simulink library "sensor_library"  (R2018b)
settings: Solver=VariableStepAuto  StartTime=0.0  StopTime=10.0  RelTol=1e-3
undefined symbols (not defined in the file): DiscIntNeverNeededParam, EOP_IERS, GPS, GPS_sensor_time, GYRO, GYRO_sensor_time, jdate0
libraries: dspsigops x26, simulink x9, simulink_extras x4
(part 2 of 2)

== matlab function sensor_library/GPS Model - [m, m//s]/GPS Clock ==
  data: jdutc input; jdut1 output; dut1 input; dat input; utc output; gps_reference output; time_error input; offset output; utc_offset output
%GPS Clock from time_convert
function [jdut1,utc,gps_reference,offset,utc_offset]= time_convert(jdutc, dut1, dat, time_error)

% ---- convert time
% Input Julian is in UTC
% UTC = UT1 - dUT1
% UT1 = UTC + dUT1
% TAI = UTC + dAT
% GPS = TAI - 19s
% TT  = GPS + 19s + 32.184s

% jdut1: is the real time to perform conversion (No error is applied)
% utc: is the estimated utc time [year,mon,day,hr,min,sec] (including time error)
% gps_reference: is the estimated gps reference time (including time error)
% offset: Receiver clock offset in seconds from GPS system time.
% utc_offset: the offset of GPS system time from UTC time, computed using almanac parameters.


% GPS reference time is the receiver’s estimate of the true GPS system time. 
% GPS reference time can be found in the header of the TIME log. 
% The relationship between GPS reference time and true GPS system time is:
% GPS system time = GPS reference time - offset


% UTC time is GPS reference time plus the current UTC offset minus the receiver clock offset
% UTC time = GPS reference time - offset + UTC offset

% ------------------------  implementation   ------------------
jdutcint=fix(jdutc);
jdutfrac=rem(jdutc,1);


%%%%%%%%%%%%%%%%%%%%%% utc
[year,mon,day,hr,min,sec] = invjday_s (jdutcint, jdutfrac);
utc_hms = hms2sec_s(hr, min, sec );

%%%%%%%%%%%%%%%%%%%%%% ut1
ut1_hms= utc_hms + dut1;
[hrtemp,mintemp,sectemp] = sec2hms_s(ut1_hms);
[jdut1int, jdut1frac] = jday_s(year,mon,day, hrtemp, mintemp, sectemp );
jdut1=jdut1int+jdut1frac;

%%%%%%%%%%%%%%%%%%%%%% output utc
utc=[year,mon,day,hr,min,sec+time_error];

%%%%%%%%%%%%%%%%%%%%%% tai
tai_hms= utc_hms + dat + time_error;

%%%%%%%%%%%%%%%%%%%%%% gps
gps_hms= tai_hms - 19; %sec
[hrtemp,mintemp,sectemp] = sec2hms_s(gps_hms);
[jdgpsint, jdgpsfrac] = jday_s(year,mon,day, hrtemp, mintemp, sectemp );
jdgps=jdgpsint+jdgpsfrac;
jdgps0 = 2.444244500000000e+06; %juliandate(1980,1,6);    % beginning of GPS week numbering
nweek = fix((jdgps-jdgps0)/7);
sow = (jdgps - (jdgps0+nweek*7)) * 3600*24;
% check sow
if sow > 604800
    nweek = nweek + 1;
    sow = sow - 604800;
elseif sow < 0
    nweek = nweek - 1;
    sow = sow + 604800;
end
gps_reference=[nweek,sow];

%%%%%%%%%%%%%%%%%%%%%% offset
offset = time_error; %To be calibrated - Now assumed to be equal to time accuracy, in order to retrieve real time
utc_offset= utc_hms - gps_hms + offset;   %UTC offset = UTC time - GPS reference time + offsert 

end

% -----------------------------------------------------------------------------
%
%                           function jday.m
%

function [jd, jdfrac] = jday_s(yr, mon, day, hr, min, sec)

% ------------------------  implementation   ------------------
jd = 367.0 * yr  ...
    - floor( (7 * (yr + floor( (mon + 9) / 12.0) ) ) * 0.25 )   ...
    + floor( 275 * mon / 9.0 ) ...
    + day + 1721013.5;   % use - 678987.0 to go to mjd directly
jdfrac = (sec + min * 60.0 + hr *3600.0) / 86400.0;

% check jdfrac
if jdfrac > 1.0
    jd = jd + floor(jdfrac);
    jdfrac = jdfrac - floor(jdfrac);
end

%  - 0.5 * sign(100.0 * yr + mon - 190002.5) + 0.5;
end

% -----------------------------------------------------------------------------
%
%                           function invjday.m
%


function [year,mon,day,hr,min,sec] = invjday_s (jd, jdfrac)

% check jdfrac for multiple days
if abs(jdfrac) >= 1.0
    jd = jd + floor(jdfrac);
    jdfrac = jdfrac - floor(jdfrac);
end

% check for fraction of a day included in the jd
dt = jd - floor(jd) - 0.5;
if (abs(dt) > 0.00000001)
    jd = jd - dt;
    jdfrac = jdfrac + dt;
end

% ----------------- find year and days of the year ---------------
temp   = jd - 2415019.5;
tu     = temp / 365.25;
year   = 1900 + floor( tu );
leapyrs= floor( ( year-1901 )*0.25 );
days   = floor(temp - ((year-1900)*365.0 + leapyrs ));

% ------------ check for case of beginning of a year -------------
if days + jdfrac < 1.0
    year   = year - 1;
    leapyrs= floor( ( year-1901 )*0.25 );
    days   = floor(temp - ((year-1900)*365.0 + leapyrs ));
end

% ------------------- find remaining data  -----------------------
% now add the daily time in to preserve accuracy
[mon,day,hr,min,sec] = days2mdh_s(year, days + jdfrac);
end

% -----------------------------------------------------------------------------
%
%                           function sec2hms
%
function [hr,min,sec] = sec2hms_s(utsec)

% ------------------------  implementation   ------------------
temp  = utsec / 3600.0;
hr    = fix( temp );
min   = fix( (temp - hr)* 60.0 );
sec   = (temp - hr - min/60.0 ) * 3600.0;
end

% -----------------------------------------------------------------------------
%
%                           function hms2sec
%
function [utsec] = hms2sec_s(hr,min,sec )

% ------------------------  implementation   ------------------
utsec  = hr * 3600.0 + min * 60.0 + sec;

end



% -----------------------------------------------------------------------------
%
%                           function days2mdh
%
function [mon,day,hr,minute,sec] = days2mdh_s (year,days)

% --------------- set up array of days in month  --------------
lmonth=zeros(12,1);
for i= 1 : 12
    lmonth(i) = 31;
    if i == 2
        lmonth(i)= 28;
    end
    if i == 4 || i == 6 || i == 9 || i == 11
        lmonth(i)= 30;
    end
end

dayofyr= floor(days);

% ----------------- find month and day of month ---------------
if rem(year-1900,4) == 0
    lmonth(2)= 29;
end

i= 1;
inttemp= 0;
while ( dayofyr > inttemp + lmonth(i) ) && ( i < 12 )
    inttemp= inttemp + lmonth(i);
    i= i+1;
end

mon= i;
day= dayofyr - inttemp;

% ----------------- find hours minutes and seconds ------------
temp = (days - dayofyr )*24.0;
hr  = fix( temp );
temp = (temp-hr) * 60.0;
minute = fix( temp );
sec = (temp-minute) * 60.0;
end

== matlab function sensor_library/GPS Model - [m, m//s]/ECI to ECEF [m,m//s] ==
  data: reci input; recef output; veci input; jdut1 input; dutt input; lod input; xp input; yp input; ddpsi input; ddeps input; vecef output
% ECI to ECEF from eci2ecef_s
% I/O - [m, m/s]

function [recef,vecef] = eci2ecef_s(reci,veci,jdut1,dutt,lod,xp,yp,ddpsi,ddeps)

eqeterms=2;
reci=reshape(reci,3,1);
veci=reshape(veci,3,1);

% ---- convert time
% Input Julian is in UT1
% UTC = UT1+dUT1
% TAI = UTC + dAT
% TT  = TAI + 32.184s
jdutt=jdut1+(dutt/24/60/60);

% Julian centuries from J2000.0
ttt=(jdutt-2451545.0)/36525;

% ---- find matrices
[prec] = precess_s(ttt);

[deltapsi,~,meaneps,omega,nut] = nutation_s(ttt,ddpsi,ddeps);

[st] = sidereal_s(jdut1,deltapsi,meaneps,omega,eqeterms );

[pm] = polarm_s(xp,yp);

% ---- perform transformations
thetasa= 7.29211514670698e-05 * (1.0  - lod/86400.0 );
omegaearth = [0; 0; thetasa;];

rpef  = st'*nut'*prec'*reci;
recef = pm'*rpef;

vpef  = st'*nut'*prec'*veci - cross( omegaearth,rpef );
vecef = pm'*vpef;

end

% -----------------------------------------------------------------------------
%
%                           function precess

function prec = precess_s (ttt)

prec=zeros(3,3);

% " to rad
convrt = pi / (180.0*3600.0);
ttt2= ttt * ttt;
ttt3= ttt2 * ttt;

% ------------------- fk4 b1980 precession angles --------------------
zeta =             2306.2181*ttt + 0.30188*ttt2 + 0.017998*ttt3; % "
theta=             2004.3109*ttt - 0.42665*ttt2 - 0.041833*ttt3;
z    =             2306.2181*ttt + 1.09468*ttt2 + 0.018203*ttt3;
% ------------------ iau 03 precession angles -------------------

zeta = zeta  * convrt;
theta= theta * convrt;
z    = z     * convrt;

% Compute COS/SIN
coszeta  = cos(zeta);
sinzeta  = sin(zeta);
costheta = cos(theta);
sintheta = sin(theta);
cosz     = cos(z);
sinz     = sin(z);

% ----------------- form matrix  mod to j2000 -----------------
prec(1,1) =  coszeta * costheta * cosz - sinzeta * sinz;
prec(1,2) =  coszeta * costheta * sinz + sinzeta * cosz;
prec(1,3) =  coszeta * sintheta;
prec(2,1) = -sinzeta * costheta * cosz - coszeta * sinz;
prec(2,2) = -sinzeta * costheta * sinz + coszeta * cosz;
prec(2,3) = -sinzeta * sintheta;
prec(3,1) = -sintheta * cosz;
prec(3,2) = -sintheta * sinz;
prec(3,3) =  costheta;

end

% -----------------------------------------------------------------------------
%
%                           function nutation

function [deltapsi, trueeps, meaneps, omega,nut] = nutation_s(ttt, ddpsi, ddeps)

nut=zeros(3,3);

deg2rad = pi/180.0;

%[iar80,rar80] = iau80in;  % coeff in deg
iar80 = ...
    [0     0     0     0     1
    0     0     2    -2     2
    0     0     2     0     2
    0     0     0     0     2
    0     1     0     0     0
    1     0     0     0     0
    0     1     2    -2     2
    0     0     2     0     1
    1     0     2     0     2
    0    -1     2    -2     2
    1     0     0    -2     0
    0     0     2    -2     1
    -1     0     2     0     2
    1     0     0     0     1
    0     0     0     2     0
    -1     0     2     2     2
    -1     0     0     0     1
    1     0     2     0     1
    2     0     0    -2     0
    -2     0     2     0     1
    0     0     2     2     2
    2     0     2     0     2
    2     0     0     0     0
    1     0     2    -2     2
    0     0     2     0     0
    0     0     2    -2     0
    -1     0     2     0     1
    0     2     0     0     0
    0     2     2    -2     2
    -1     0     0     2     1
    0     1     0     0     1
    1     0     0    -2     1
    0    -1     0     0     1
    2     0    -2     0     0
    -1     0     2     2     1
    1     0     2     2     2
    0    -1     2     0     2
    0     0     2     2     1
    1     1     0    -2     0
    0     1     2     0     2
    -2     0     0     2     1
    0     0     0     2     1
    2     0     2    -2     2
    1     0     0     2     0
    1     0     2    -2     1
    0     0     0    -2     1
    0    -1     2    -2     1
    2     0     2     0     1
    1    -1     0     0     0
    1     0     0    -1     0
    0     0     0     1     0
    0     1     0    -2     0
    1     0    -2     0     0
    2     0     0    -2     1
    0     1     2    -2     1
    1     1     0     0     0
    1    -1     0    -1     0
    -1    -1     2     2     2
    0    -1     2     2     2
    1    -1     2     0     2
    3     0     2     0     2
    -2     0     2     0     2
    1     0     2     0     0
    -1     0     2     4     2
    1     0     0     0     2
    -1     0     2    -2     1
    0    -2     2    -2     1
    -2     0     0     0     1
    2     0     0     0     1
    3     0     0     0     0
    1     1     2     0     2
    0     0     2     1     2
    1     0     0     2     1
    1     0     2     2     1
    1     1     0    -2     1
    0     1     0     2     0
    0     1     2    -2     0
    0     1    -2     2     0
    1     0    -2     2     0
    1     0    -2    -2     0
    1     0     2    -2     0
    1     0     0    -4     0
    2     0     0    -4     0
    0     0     2     4     2
    0     0     2    -1     2
    -2     0     2     4     2
    2     0     2     2     2
    0    -1     2     0     1
    0     0    -2     0     1
    0     0     4    -2     2
    0     1     0     0     2
    1     1     2    -2     2
    3     0     2    -2     2
    -2     0     2     2     2
    -1     0     0     0     2
    0     0    -2     2     1
    0     1     2     0     1
    -1     0     4     0     2
    2     1     0    -2     0
    2     0     0     2     0
    2     0     2    -2     1
    2     0    -2     0     1
    1    -1     0    -2     0
    -1     0     0     1     1
    -1    -1     0     2     1
    0     1     0     1     0];

rar80 = 1.0e-04 * ...
    [-0.833860138961157  -0.000844545432493   0.446149790041050   0.000043148417619
    -0.063932380127915  -0.000007757018898   0.027808912748443  -0.000015029224114
    -0.011024663108431  -0.000000969627362   0.004736629664440  -0.000002424068406
    0.009996858104479   0.000000969627362  -0.004339082445930   0.000002424068406
    0.006913443092622  -0.000016483665158   0.000261799387799  -0.000000484813681
    0.003451873409500   0.000000484813681  -0.000033936957678                   0
    -0.002506486731336   0.000005817764173   0.001085982645685  -0.000002908882087
    -0.001871380809083  -0.000001939254724   0.000969627362219                   0
    -0.001459289180140                   0   0.000625409648631  -0.000000484813681
    0.001052045688008  -0.000002424068406  -0.000460572997054   0.000001454441043
    -0.000766005616153                   0  -0.000004848136811                   0
    0.000625409648631   0.000000484813681  -0.000339369576777                   0
    0.000596320827765                   0  -0.000256951250988                   0
    0.000305432619099   0.000000484813681  -0.000159988514766                   0
    0.000305432619099                   0  -0.000009696273622                   0
    -0.000286040071855                   0   0.000126051557088                   0
    -0.000281191935044  -0.000000484813681   0.000155140377955                   0
    -0.000247254977366                   0   0.000130899693900                   0
    0.000232710566933                   0   0.000004848136811                   0
    0.000223014293310                   0  -0.000116355283466                   0
    -0.000184229198822                   0   0.000077570188978                   0
    -0.000150292241144                   0   0.000063025778544                   0
    0.000140595967522                   0  -0.000004848136811                   0
    0.000140595967522                   0  -0.000058177641733                   0
    0.000126051557088                   0  -0.000004848136811                   0
    -0.000106659009844                   0                   0                   0
    0.000101810873033                   0  -0.000048481368111                   0
    0.000082418325789  -0.000000484813681                   0                   0
    -0.000077570188978   0.000000484813681   0.000033936957678                   0
    0.000077570188978                   0  -0.000038785094489                   0
    -0.000072722052166                   0   0.000043633231300                   0
    -0.000063025778544                   0   0.000033936957678                   0
    -0.000058177641733                   0   0.000029088820867                   0
    0.000053329504922                   0                   0                   0
    -0.000048481368111                   0   0.000024240684055                   0
    -0.000038785094489                   0   0.000014544410433                   0
    -0.000033936957678                   0   0.000014544410433                   0
    -0.000033936957678                   0   0.000014544410433                   0
    -0.000033936957678                   0                   0                   0
    0.000033936957678                   0  -0.000014544410433                   0
    -0.000029088820867                   0   0.000014544410433                   0
    -0.000029088820867                   0   0.000014544410433                   0
    0.000029088820867                   0  -0.000014544410433                   0
    0.000029088820867                   0                   0                   0
    0.000029088820867                   0  -0.000014544410433                   0
    -0.000024240684055                   0   0.000014544410433                   0
    -0.000024240684055                   0   0.000014544410433                   0
    -0.000024240684055                   0   0.000014544410433                   0
    0.000024240684055                   0                   0                   0
    -0.000019392547244                   0                   0                   0
    -0.000019392547244                   0                   0                   0
    -0.000019392547244                   0                   0                   0
    0.000019392547244                   0                   0                   0
    0.000019392547244                   0  -0.000009696273622                   0
    0.000019392547244                   0  -0.000009696273622                   0
    -0.000014544410433                   0                   0                   0
    -0.000014544410433                   0                   0                   0
    -0.000014544410433                   0   0.000004848136811                   0
    -0.000014544410433                   0   0.000004848136811                   0
    -0.000014544410433                   0   0.000004848136811                   0
    -0.000014544410433                   0   0.000004848136811                   0
    -0.000014544410433                   0   0.000004848136811                   0
    0.000014544410433                   0                   0                   0
    -0.000009696273622                   0   0.000004848136811                   0
    -0.000009696273622                   0   0.000004848136811                   0
    -0.000009696273622                   0   0.000004848136811                   0
    -0.000009696273622                   0   0.000004848136811                   0
    -0.000009696273622                   0   0.000004848136811                   0
    0.000009696273622                   0  -0.000004848136811                   0
    0.000009696273622                   0                   0                   0
    0.000009696273622                   0  -0.000004848136811                   0
    0.000009696273622                   0  -0.000004848136811                   0
    -0.000004848136811                   0                   0                   0
    -0.000004848136811                   0   0.000004848136811                   0
    -0.000004848136811                   0                   0                   0
    -0.000004848136811                   0                   0                   0
    -0.000004848136811                   0                   0                   0
    -0.000004848136811                   0                   0                   0
    -0.000004848136811                   0                   0                   0
    -0.000004848136811                   0                   0                   0
    -0.000004848136811                   0                   0                   0
    -0.000004848136811                   0                   0                   0
    -0.000004848136811                   0                   0                   0
    -0.000004848136811                   0                   0                   0
    -0.000004848136811                   0                   0                   0
    -0.000004848136811                   0   0.000004848136811                   0
    -0.000004848136811                   0                   0                   0
    -0.000004848136811                   0                   0                   0
    -0.000004848136811                   0                   0                   0
    0.000004848136811                   0                   0                   0
    0.000004848136811                   0                   0                   0
    0.000004848136811                   0  -0.000004848136811                   0
    0.000004848136811                   0                   0                   0
    0.000004848136811                   0  -0.000004848136811                   0
    0.000004848136811                   0  -0.000004848136811                   0
    0.000004848136811                   0                   0                   0
    0.000004848136811                   0                   0                   0
    0.000004848136811                   0                   0                   0
    0.000004848136811                   0                   0                   0
    0.000004848136811                   0                   0                   0
    0.000004848136811                   0  -0.000004848136811                   0
    0.000004848136811                   0                   0                   0
    0.000004848136811                   0                   0                   0
    0.000004848136811                   0                   0                   0
    0.000004848136811                   0                   0                   0
    0.000004848136811                   0                   0                   0];

% ---- determine coefficients for iau 1980 nutation theory ----
ttt2= ttt*ttt;
ttt3= ttt2*ttt;

meaneps = -46.8150 *ttt - 0.00059 *ttt2 + 0.001813 *ttt3 + 84381.448;
meaneps = rem( meaneps/3600.0, 360.0 );
meaneps = meaneps * deg2rad;

[l, l1, f, d, omega] = fundarg_s(ttt);

deltapsi= 0.0;
deltaeps= 0.0;
for i= 106:-1: 1
    tempval= iar80(i,1)*l + iar80(i,2)*l1 + iar80(i,3)*f + ...
        iar80(i,4)*d + iar80(i,5)*omega;
    deltapsi= deltapsi + (rar80(i,1)+rar80(i,2)*ttt) * sin( tempval );
    deltaeps= deltaeps + (rar80(i,3)+rar80(i,4)*ttt) * cos( tempval );
end

% --------------- find nutation parameters --------------------
deltapsi = rem( deltapsi + ddpsi, 2.0 * pi );
deltaeps = rem( deltaeps + ddeps, 2.0 * pi );
trueeps  = meaneps + deltaeps;

cospsi  = cos(deltapsi);
sinpsi  = sin(deltapsi);
coseps  = cos(meaneps);
sineps  = sin(meaneps);
costrueeps = cos(trueeps);
sintrueeps = sin(trueeps);

nut(1,1) =  cospsi;
nut(1,2) =  costrueeps * sinpsi;
nut(1,3) =  sintrueeps * sinpsi;
nut(2,1) = -coseps * sinpsi;
nut(2,2) =  costrueeps * coseps * cospsi + sintrueeps * sineps;
nut(2,3) =  sintrueeps * coseps * cospsi - sineps * costrueeps;
nut(3,1) = -sineps * sinpsi;
nut(3,2) =  costrueeps * sineps * cospsi - sintrueeps * coseps;
nut(3,3) =  sintrueeps * sineps * cospsi + costrueeps * coseps;

end

% -----------------------------------------------------------------------------
%
%                           function fundarg

function [ l, l1, f, d, omega] = fundarg_s(ttt)

deg2rad = pi/180.0;

% ---- determine coefficients for iau 1980 nutation theory ----
l = ((((0.064) * ttt + 31.310) * ttt + 1717915922.6330) * ttt) / 3600.0 + 134.96298139;
l1 = ((((-0.012) * ttt - 0.577) * ttt + 129596581.2240) * ttt) / 3600.0 + 357.52772333;
f = ((((0.011) * ttt - 13.257) * ttt + 1739527263.1370) * ttt) / 3600.0 + 93.27191028;
d = ((((0.019) * ttt - 6.891) * ttt + 1602961601.3280) * ttt) / 3600.0 + 297.85036306;
omega = ((((0.008) * ttt + 7.455) * ttt - 6962890.5390) * ttt) / 3600.0 + 125.04452222;

% ---- convert units to rad
l    = rem( l,360.0  )     * deg2rad; % rad
l1   = rem( l1,360.0  )    * deg2rad;
f    = rem( f,360.0  )     * deg2rad;
d    = rem( d,360.0  )     * deg2rad;
omega= rem( omega,360.0  ) * deg2rad;

end

% -----------------------------------------------------------------------------
%
%                           function sidereal

function [st]  = sidereal_s(jdut1, deltapsi, meaneps, omega, eqeterms )

st=zeros(3,3);

% ------------------------ find gmst --------------------------
gmst= gstime_s(jdut1);

% ------------------------ find mean ast ----------------------
% after 1997, kinematic terms apply as well as gemoetric in eqe
if (jdut1 > 2450449.5 ) && (eqeterms > 0)
    ast= gmst + deltapsi* cos(meaneps) ...
        + 0.00264*pi /(3600*180)*sin(omega) ...
        + 0.000063*pi /(3600*180)*sin(2.0 *omega);
else
    ast= gmst + deltapsi* cos(meaneps);
end

ast = rem (ast, 2.0*pi);

st(1,1) =  cos(ast);
st(1,2) = -sin(ast);
st(1,3) =  0.0;
st(2,1) =  sin(ast);
st(2,2) =  cos(ast);
st(2,3) =  0.0;
st(3,1) =  0.0;
st(3,2) =  0.0;
st(3,3) =  1.0;

end

% -----------------------------------------------------------------------------
%
%                           function gstime

function gst = gstime_s(jdut1)

twopi      = 2.0*pi;
deg2rad    = pi/180.0;

% ------------------------  implementation   ------------------
tut1= ( jdut1 - 2451545.0 ) / 36525.0;

temp = - 6.2e-6 * tut1 * tut1 * tut1 + 0.093104 * tut1 * tut1  ...
    + (876600.0 * 3600.0 + 8640184.812866) * tut1 + 67310.54841;

% 360/86400 = 1/240, to deg, to rad
temp = rem( temp*deg2rad/240.0,twopi );

% ------------------------ check quadrants --------------------
if ( temp < 0.0 )
    temp = temp + twopi;
end

gst = temp;
end

% -----------------------------------------------------------------------------
%
%                           function polarm

function [pm] = polarm_s (xp, yp)

pm=zeros(3,3);

cosxp = cos(xp);
sinxp = sin(xp);
cosyp = cos(yp);
sinyp = sin(yp);

pm(1,1) =  cosxp;
pm(1,2) =  0.0;
pm(1,3) = -sinxp;
pm(2,1) =  sinxp * sinyp;
pm(2,2) =  cosyp;
pm(2,3) =  cosxp * sinyp;
pm(3,1) =  sinxp * cosyp;
pm(3,2) = -sinyp;
pm(3,3) =  cosxp * cosyp;

end

== matlab function sensor_library/GPS Model - [m, m//s]/ECEF to LLH [rad, m] ==
  data: r_ecef input; latgc output; latgd output; lon output; hellp output
%ECEF to LLH from ecef2llh
%H ellipsoid WGS-84
%input [m]
%output [rad,rad,rad,m]

function [latgc,latgd,lon,hellp] = ecef2llh (r_ecef)
small =     1e-8;
% convert e_ecef to km
r_ecef=r_ecef./1000;
% WGS-84 Parameter
a  = 6378.137; %km
rb = 6356.752314245179; %km

% -------------------------  implementation   -------------------------
% ---------------- find longitude value  ----------------------
rd = sqrt( r_ecef(1)*r_ecef(1) + r_ecef(2)*r_ecef(2) );
if ( abs( rd ) < small )
    rtasc= sign(r_ecef(3))*pi*0.5;
else
    rtasc= atan2( r_ecef(2)/rd , r_ecef(1)/rd );
end

%Geodetic/Geocentric longitude -rad
lon  = rtasc;

% -------------- set up initial latitude value  ---------------
atemp= 1.0 /(a*rd);
b = sign(r_ecef(3)) * rb;
E= (b*r_ecef(3)-a*a+b*b)*atemp;
F= (b*r_ecef(3)+a*a-b*b)*atemp;
third= 1.0 /3.0;
P= 4.0 *third*(E*F + 1.0);
Q= 2.0 *(E*E - F*F);
D= P*P*P + Q*Q;

if ( D > 0.0  )
    NU= (sqrt(D)-Q)^third - (sqrt(D)+Q)^third;
else
    sqrtp= sqrt(-P);
    NU= 2.0 *sqrtp*cos( third*acos(Q/(P*sqrtp)) );
end
G= 0.5 *(sqrt(E*E + NU) + E);
t= sqrt(G*G + (F-NU*G)/(2.0 *G-E)) - G;

%Geodetic latitude - rad
latgd= atan(a*(1.0 -t*t)/(2.0 *b*t));

%Geocentric latitude - rad
latgc = gd2gc_s( latgd );

% Ellipsoid altitude - km
hellp= (rd-a*t)*cos( latgd) + (r_ecef(3)-b)*sin(latgd);
% Ellipsoid altitude - m
hellp=hellp*1000;

end

% -----------------------------------------------------------------------------
%
%                           function gd2gc

function [latgc] = gd2gc_s(latgd)

eesqrd = 0.006694379990141;    % WGS-84 eccentricity of earth sqrd

% -------------------------  implementation   -----------------
latgc= atan((1.0 - eesqrd)*tan(latgd) );
end
